simulink model "tst_bus_outputasbus"  (Simulink 8.0)
settings: Solver=ode45  StartTime=0.0  StopTime=10.0  RelTol=1e-3
settings Model: Creator=Marci  LastModifiedBy=Marci

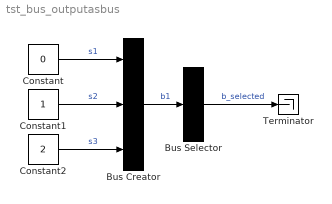
== system tst_bus_outputasbus ==
  Bus Creator : BusCreator  Inputs=3
  Bus Selector : BusSelector  OutputSignals=s2,s3  OutputAsBus=on
  Constant : Constant  Value=0
  Constant1 : Constant
  Constant2 : Constant  Value=2
  Terminator : Terminator
  wires:
  Bus Creator/1 -> Bus Selector/1  "b1"
  Constant/1 -> Bus Creator/1  "s1"
  Constant1/1 -> Bus Creator/2  "s2"
  Bus Selector/1 -> Terminator/1  "b_selected"
  Constant2/1 -> Bus Creator/3  "s3"
